simulink model "quadcopter_model_c_Euler"  (Simulink 8.7)
settings: Solver=VariableStepAuto  StartTime=0.0  StopTime=2  RelTol=1e-3
undefined symbols (not defined in the file): A, g, I, initial_eta, initial_etadot, initial_xi, initial_xidot, m
settings Model: Creator=Daniel  LastModifiedBy=mgreiff
settings DataIOCC: SaveFormat=Dataset
settings DebuggingCC: UnderspecifiedInitializationDetection=Simplified  MergeDetectMultiDrivingBlocksExec=error  AllowSymbolicDim=off
settings HardwareCC: ProdBitPerPointer=64  ProdLargestAtomicFloat=Float  ProdIntDivRoundTo=Zero  ProdEndianess=LittleEndian  ProdWordSize=64  ProdHWDeviceType=Intel->x86-64 (Windows64)
settings GRTTargetCC: GeneratePreprocessorConditionals=Use local settings
settings ConfigComp: CovModelRefEnable=off

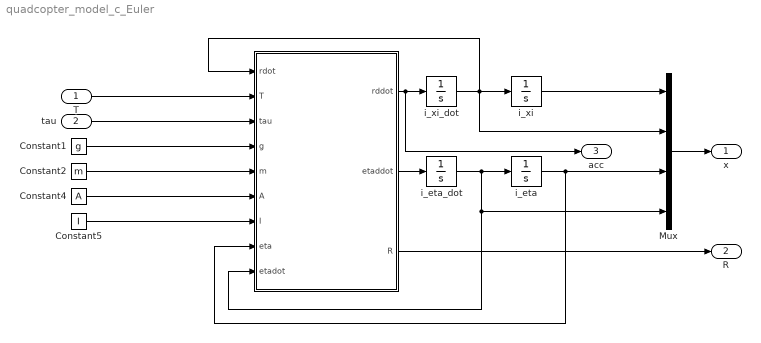
== system quadcopter_model_c_Euler ==
  T : Inport  PortDimensions=1
  tau : Inport  Port=2  PortDimensions=3
  " " : MATLAB Function  TreatAsAtomicUnit=on
  Constant1 : Constant  Value=g
  Constant2 : Constant  Value=m
  Constant4 : Constant  Value=A
  Constant5 : Constant  Value=I
  Mux : Mux
  i_eta : Integrator  InitialCondition=initial_eta
  i_eta_dot : Integrator  InitialCondition=initial_etadot
  i_xi : Integrator  InitialCondition=initial_xi
  i_xi_dot : Integrator  InitialCondition=initial_xidot
  x : Outport
  R : Outport  Port=2
  acc : Outport  Port=3
  wires:
  " "/2(etaddot) -> i_eta_dot/1
  " "/1(rddot) -> acc/1, i_xi_dot/1
  i_xi_dot/1 -> Mux/2, " "/1(rdot), i_xi/1
  i_eta_dot/1 -> i_eta/1, " "/9(etadot), Mux/4
  i_eta/1 -> " "/8(eta), Mux/3
  i_xi/1 -> Mux/1
  Constant4/1 -> " "/6(A)
  Constant2/1 -> " "/5(m)
  Constant1/1 -> " "/4(g)
  Constant5/1 -> " "/7(I)
  " "/3(R) -> R/1
  T/1 -> " "/2(T)
  Mux/1 -> x/1
  tau/1 -> " "/3(tau)

== matlab function   ==
  data: rdot input double; T input double; tau input double; g input double; m input double; A input double; I input double; rddot output double; eta input double; etadot input double; etaddot output double; R output double
function [ rddot,etaddot,R] = quad_acceleration(rdot, T, tau, g, m, A, I, eta, etadot)
    % Equations from Teppo Luukkonen, Modelling and control of quadcopter
    phi = eta(1); theta = eta(2); psi = eta(3); % Roll, pitch, yaw
    phidot = etadot(1); thetadot = etadot(2); psidot = etadot(3); % Roll, pitch, yaw
    
    % Gravity acceleration
    Ga = -g * [0; 0; 1];
    
    % Thrust acceleration
    angM = [cos(psi)*sin(theta)*cos(phi) + sin(psi)*sin(phi);
          sin(psi)*sin(theta)*cos(phi) - cos(psi)*sin(phi);
          cos(theta)*cos(phi)];
    Ta = T/m * angM;
    
    % Drag
    Aa = -1/m * diag(A) * rdot;
    
    rddot = Ga + Ta + Aa; % (21)
    
    % Define the C-matrix as (19)
    Ixx = I(1); Iyy = I(2); Izz = I(3);
    Sphi = sin(phi); Stheta = sin(theta); Spsi = sin(psi);
    Cphi = cos(phi); Ctheta = cos(theta); Cpsi = cos(psi);
    
    C11 = 0;
    C12 = (Iyy - Izz) * (thetadot*Cphi*Sphi + psidot*Sphi^2*Ctheta) + (Izz - Iyy)*psidot*Cphi^2*Ctheta - Ixx*psidot*Ctheta;
    C13 = (Izz - Iyy) * psidot*Cphi*Sphi*Ctheta^2;
    C21 = (Izz - Iyy) * (thetadot*Cphi*Sphi + psidot*Sphi*Ctheta) + (Iyy - Izz)*psidot*Cphi^2*Ctheta - Ixx*psidot*Ctheta;
    C22 = (Izz - Iyy) * phidot*Cphi*Sphi;
    C23 = -Ixx * psidot * Stheta * Ctheta + Iyy * psidot * Sphi^2 * Stheta * Ctheta + Izz * psidot * Cphi^2 * Stheta * Ctheta;
    C31 = (Iyy - Izz) * psidot * Ctheta^2 * Sphi * Cphi - Ixx * thetadot * Ctheta;
    C32 = (Izz - Iyy) * (thetadot * Cphi * Sphi * Stheta + phidot * Sphi^2 * Ctheta) + (Iyy - Izz) * phidot * Cphi^2 * Ctheta...
            + Ixx * psidot * Stheta * Ctheta - Iyy * psidot * Sphi^2 * Stheta * Ctheta - Izz * psi * Cphi^2 * Stheta * Ctheta;
    C33 = (Iyy - Izz) * phidot * Cphi * Sphi * Ctheta^2 - Iyy * thetadot * Sphi^2 * Ctheta * Stheta ...
            - Izz * thetadot * Cphi^2 * Ctheta * Stheta + Ixx * thetadot * Ctheta * Stheta;
    
    C = [C11 C12 C13; C21 C22 C23; C31 C32 C33];

    % (16)
    J11 = Ixx; J12 = 0; J13 = -Ixx*Stheta;
    J21 = 0;
    J22 = Iyy * Cphi^2 + Izz * Sphi^2;
    J23 = (Iyy - Izz) * Cphi * Sphi * Ctheta;
    J31 = -Ixx * Stheta;
    J32 = (Iyy - Izz)*Cphi*Sphi*Ctheta;
    J33 = Ixx * Stheta^2 + Iyy * Sphi^2 * Ctheta^2 + Izz * Cphi^2*Ctheta^2;
    J = [J11 J12 J13; J21 J22 J23; J31 J32 J33];  
    
    persistent etadotm1
    if isempty(etadotm1)
        etadotm1 = zeros(3,1);
    end
    lim = 0.1;
    if abs(Cphi) < lim || abs(Ctheta) < lim
        etaddot = etadotm1;
    else
        etaddot = J\(tau - C*etadot); % (20)
    end
    etadotm1 = etaddot;

    R = [Cpsi*Ctheta, Cpsi*Stheta*Sphi-Spsi*Cphi, Cpsi*Stheta*Cphi + Spsi*Sphi;
        Spsi*Ctheta, Spsi*Stheta*Sphi+Cpsi*Cphi, Spsi*Stheta*Cphi - Cpsi*Sphi;
        -Stheta, Ctheta*Sphi, Ctheta*Cphi];
end
